simulink model "single_area_model_PI_control"  (R2014b)
settings: Solver=ode45  StartTime=0.0  StopTime=11.0  RelTol=1e-3
settings Model: Creator=Shane Reynolds  LastModifiedBy=Shane Reynolds

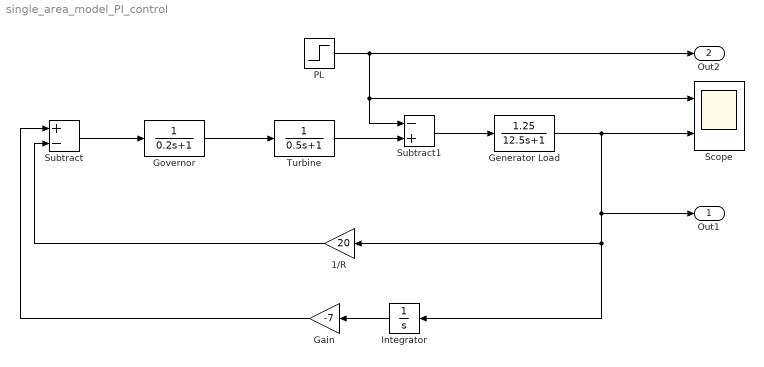
== system single_area_model_PI_control ==
  1/R : Gain  Gain=20
  Gain : Gain  Gain=-7
  Generator Load : TransferFcn  Numerator=[1.25]  Denominator=[12.5 1]
  Governor : TransferFcn  Denominator=[0.2 1]
  Integrator : Integrator
  PL : Step  After=0.2  SampleTime=0
  Scope : Scope  NumInputPorts=2
      settings: YMin=-1~-1  YMax=1~1
  Subtract : Sum  Inputs=+-
  Subtract1 : Sum  Inputs=-+
  Turbine : TransferFcn  Denominator=[0.5 1]
  Out1 : Outport
  Out2 : Outport  Port=2
  wires:
  Governor/1 -> Turbine/1
  Subtract/1 -> Governor/1
  1/R/1 -> Subtract/2
  Turbine/1 -> Subtract1/2
  Subtract1/1 -> Generator Load/1
  PL/1 -> Scope/1, Subtract1/1, Out2/1
  Generator Load/1 -> Scope/2, Out1/1, Integrator/1, 1/R/1
  Integrator/1 -> Gain/1
  Gain/1 -> Subtract/1
